simulink model "prob_15a"  (R2015a)
settings: Solver=ode45  StartTime=0.0  StopTime=24  RelTol=1e-3
settings Model: Creator=Anu  LastModifiedBy=Anu

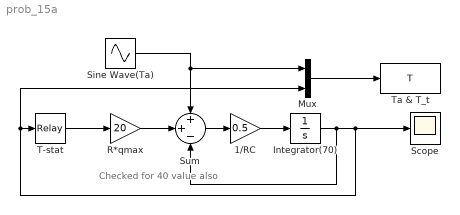
== system prob_15a ==
  note: Checked for 40
      |     value also
  1/RC : Gain  Gain=0.5
  Integrator(70) : Integrator  InitialCondition=70
  Mux : Mux  Inputs=2
  R*qmax : Gain  Gain=20
  Scope : Scope
  Sine Wave(Ta) : Sin  Amplitude=10  Bias=50  Frequency=pi/12  SampleTime=0
  Sum : Sum  Inputs=++-
  T-stat : Relay  OnSwitchValue=71  OffSwitchValue=69  OnOutputValue=0  OffOutputValue=1
  Ta & T_t : ToWorkspace  VariableName=T  SampleTime=-1
  wires:
  T-stat/1 -> R*qmax/1
  R*qmax/1 -> Sum/2
  Sum/1 -> 1/RC/1
  1/RC/1 -> Integrator(70)/1
  Integrator(70)/1 -> Sum/3, Mux/2, T-stat/1, Scope/1
  Sine Wave(Ta)/1 -> Mux/1, Sum/1
  Mux/1 -> Ta & T_t/1
